simulink model "step2berevm"  (R2015a)
settings: Solver=ode45  StartTime=0.0  StopTime=1  RelTol=1e-3
values from neighbouring files (symbols this model uses):
  Dt = 1/(SampleRate*(N_in/N_out))    [DVBs2.m]    (also in DVBs2_2.m; Script.m)
  K_BCH = 51648    [DVBs2.m]    (also in DVBs2_2.m; Script.m)
  N_in = BBHEADER + DFL    [DVBs2.m]    (also in DVBs2_2.m; Script.m)
  Poly_ampl = polyfit(Xampl_0,DPDampl_0,PolyOrder)    [step1func.m]
  Poly_phase = polyfit(Xampl_0,DPDphase_0,PolyOrder)    [step1func.m]
  roll_off = 0.25    [DVBs2.m]    (also in DVBs2_2.m; Script.m)
undefined symbols (not defined in the file or in its folder): gcbh, rcfiltgaincompat
libraries: commblkcod2 x4, commfilt2 x3, commutil2 x2, dsppolyfun x2, dspsigops x2, commsequence2 x2, commdigbbndam3 x2, commblkintrlv2 x2, commchan3 x1, commrflib2 x1, commrandsrc2 x1, commsink2 x1
settings Model: Creator=Study  LastModifiedBy=Наталья
settings DataIOCC: SignalLoggingSaveFormat=ModelDataLogs
settings DebuggingCC: FcnCallInpInsideContextMsg=UseLocalSettings
settings GRTTargetCC: CombineOutputUpdateFcns=off  GRTInterface=on

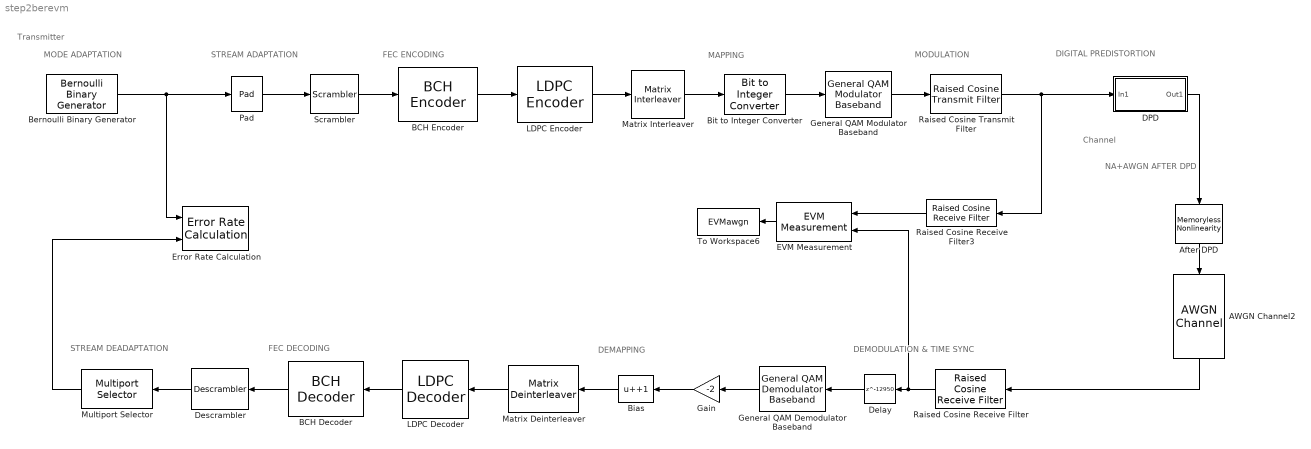
== system step2berevm ==
  note: DIGITAL PREDISTORTION
  note: DEMODULATION & TIME SYNC
  note: DEMAPPING
  note: FEC DECODING
  note: STREAM DEADAPTATION
  note: NA+AWGN
      | AFTER DPD
  note: Channel
  note: MODULATION
  note: MAPPING
  note: FEC ENCODING
  note: STREAM ADAPTATION
  note: MODE ADAPTATION
  note: Transmitter
  AWGN Channel2 : commchan3/AWGN Channel  InputProcessing=Columns as channels (frame based)  seed=67  noiseMode="Signal to noise ratio  (SNR)"  EbNodB=10  EsNodB=10  SNRdB=SNR  bitsPerSym=1  Ps=0.2562  Tsym=1  variance=1
  After DPD : commrflib2/Memoryless Nonlinearity  model_select=Saleh model  linGaindB=0  GindB=0  iip3=30  am2pm=10  LPwrLimAMPM=10  UPwrLimAMPM=inf  amam=AM_AM  ampm=AM_PM  x=[8.1081 1.5413 6.5202 -0.0718]  y=[4.6645 2.0965 10.88 -0.003]  p=0.5  GoutdB=0  vsat=1
  BCH Decoder : commblkcod2/BCH Decoder  n=N_BCH  k=K_BCH  specShortening=off  shortenedK=5  specGenPoly=on  genPoly=BCHGeneratorPoly  specPrimPoly=on  prPoly=BCHPrimitivePoly  specDisableGenCheck=off  specPuncture=off  punctVec=[ones(8,1); zeros(2,1)]  specErasurePort=off  showNumErr=off
  BCH Encoder : commblkcod2/BCH Encoder  n=N_BCH  k=K_BCH  specShortening=off  shortenedK=5  specGenPoly=on  genPoly=BCHGeneratorPoly  specPrimPoly=on  prPoly=BCHPrimitivePoly  specDisableGenCheck=off  specPuncture=off  punctVec=[ones(8,1); zeros(2,1)]
  Bernoulli Binary Generator : commrandsrc2/Bernoulli Binary Generator  P=0.5  seed=61  Ts=Dt  frameBased=on  sampPerFrame=N_in  orient=off  outDataType=double
  Bias : Bias  Bias=+1
  Bit to Integer Converter : commutil2/Bit to Integer Converter  nbits=NMOD  bitOrder=MSB first  signedOutputValues=Unsigned  outDtype=Inherit via internal rule  outDtypeSigned=Inherit via internal rule
  DPD : Subsystem
  Delay : Delay  DelayLength=12950  InitialCondition=0  InputProcessing=Columns as channels (frame based)
  Descrambler : commsequence2/Descrambler  M=2  poly=[1 0 0 0 0 0 0 0 0 0 0 0 0 0 1 1]  iniStaSource=Dialog Parameter  ini_sta=[1 0 0 1 0 1 0 1 0 0 0 0 0 0 0]  resetViaPort=off
  EVM Measurement : commutil2/EVM Measurement  normMethod=Average reference signal power  averagePower=1  peakPower=1  maxOrMinOut=off  percentileOut=off  percentileVal=95  nSym=off
  Error Rate Calculation : commsink2/Error Rate Calculation  N=N_in  st_delay=100  cp_mode=Entire frame  subframe=[]  PMode=Workspace  WsName=BERawgn  RsMode2=off  stop=off  numErr=100  maxBits=1e6
  Gain : Gain  Gain=-2
  General QAM Demodulator Baseband : commdigbbndam3/General QAM Demodulator Baseband  SigCon=apsk32  OutType=Bit  DecType=Hard decision  VarSource=Dialog  Variance=1  outDtypeBit=Inherit via internal rule  outDtype=Inherit via internal rule  roundingMode=Floor  overflowMode=Wrap  sigConstWordLen=16  accum1WordLen=32  accum1FracLen=30  prodInWordLen=32  prodInFracLen=30  prodOutWordLen=32  prodOutFracLen=30  accum2WordLen=32  accum2FracLen=30  accum3WordLen=32  accum3FracLen=30  nsiWordLen=32  nsiFracLen=30  invn0WordLen=16  invn0FracLen=8  outputWordLen=32  outputFracLen=30
  General QAM Modulator Baseband : commdigbbndam3/General QAM Modulator Baseband  SigCon=apsk32  outDtype=double  outWordLen=16  outUDDataType=sfix(16)  outFracLenMode=Best precision  outFracLen=15
  LDPC Decoder : commblkcod2/LDPC Decoder  ParityCheckMat=H  OutputFmt=Information part  DecisionType=Hard decision  OutputDataType=double  NumIter=50  DoParityCheck=on  OutputNumIter=off  OutputFinalChecks=off
  LDPC Encoder : commblkcod2/LDPC Encoder  ParityCheckMat=H
  Matrix Deinterleaver : commblkintrlv2/Matrix Deinterleaver  Nrows=Numofcols  Ncols=Numofrows
  Matrix Interleaver : commblkintrlv2/Matrix Interleaver  Nrows=Numofcols  Ncols=Numofrows
  Multiport Selector : dspindex/Multiport Selector  rowsOrCols=Rows  idxCellArray=[1:N_in]  idxErrMode=Clip Index
  Pad : dspsigops/Pad  padAlong=Columns  dimsToPad=1  valSrc=Specify via dialog  padVal=0  spec=Output size  padNumOutRowsSpecMethod=User-specified  numOutRows=K_BCH  padNumOutColsSpecMethod=User-specified  numOutCols=1  isVarDimsMode=off  padBeginning=0  padEnd=0  outSizeMode=User-specified  outSize=1  padSigAt=End  trunc_flag=None  roundingMode=Floor  overflowMode=off  truncOrWrapMode=Truncate  wrap_flag=None
  Raised Cosine Receive Filter : commfilt2/Raised Cosine Receive Filter  filtType=Square root  N=8  filtSpan=2*(10)/2  currentFiltSpan=2*(10)/2  D=(2*(10)/2)/2  R=roll_off  sampMode=Mute  saveAsFlag=0  rateMode=Downsampling  downFactor=8  downOffset=0  framing=Enforce single-rate processing  InputProcessing=Columns as channels (frame based)  checkGain=Normalized  filterGain=rcfiltgaincompat(gcbh)  checkCoeff=off  variableName=rcRxFilt  launchFVT=off  roundingMode=Floor  overflowMode=off
  Raised Cosine Receive Filter3 : commfilt2/Raised Cosine Receive Filter  filtType=Square root  N=8  filtSpan=2*(10)/2  currentFiltSpan=2*(10)/2  D=(2*(10)/2)/2  R=roll_off  sampMode=Mute  saveAsFlag=0  rateMode=Downsampling  downFactor=8  downOffset=0  framing=Enforce single-rate processing  InputProcessing=Columns as channels (frame based)  checkGain=Normalized  filterGain=rcfiltgaincompat(gcbh)  checkCoeff=off  variableName=rcRxFilt3  launchFVT=off  roundingMode=Floor  overflowMode=off
  Raised Cosine Transmit Filter : commfilt2/Raised Cosine Transmit Filter  filtType=Square root  filtSpan=2*(10)/2  currentFiltSpan=2*(10)/2  D=(2*(10)/2)/2  R=roll_off  sampMode=Mute  saveAsFlag=0  N=8  framing=Enforce single-rate processing  InputProcessing=Columns as channels (frame based)  checkGain=Normalized  filterGain=rcfiltgaincompat(gcbh)  checkCoeff=off  variableName=rcTxFilt  launchFVT=off  roundingMode=Floor  overflowMode=off
  Scrambler : commsequence2/Scrambler  M=2  poly=[1 0 0 0 0 0 0 0 0 0 0 0 0 0 1 1]  iniStaSource=Dialog Parameter  ini_sta=[1 0 0 1 0 1 0 1 0 0 0 0 0 0 0]  resetViaPort=off
  To Workspace6 : ToWorkspace  VariableName=EVMawgn  SampleTime=-1
      settings: Save2DSignal=2-D array (concatenate along first dimension)
  wires:
  Bernoulli Binary Generator/1 -> Error Rate Calculation/1, Pad/1
  Scrambler/1 -> BCH Encoder/1
  BCH Encoder/1 -> LDPC Encoder/1
  Pad/1 -> Scrambler/1
  Matrix Interleaver/1 -> Bit to Integer Converter/1
  Bit to Integer Converter/1 -> General QAM Modulator Baseband/1
  LDPC Encoder/1 -> Matrix Interleaver/1
  General QAM Modulator Baseband/1 -> Raised Cosine Transmit Filter/1
  General QAM Demodulator Baseband/1 -> Gain/1
  Gain/1 -> Bias/1
  Bias/1 -> Matrix Deinterleaver/1
  Matrix Deinterleaver/1 -> LDPC Decoder/1
  LDPC Decoder/1 -> BCH Decoder/1
  BCH Decoder/1 -> Descrambler/1
  Descrambler/1 -> Multiport Selector/1
  Delay/1 -> General QAM Demodulator Baseband/1
  Multiport Selector/1 -> Error Rate Calculation/2
  AWGN Channel2/1 -> Raised Cosine Receive Filter/1
  Raised Cosine Receive Filter/1 -> EVM Measurement/2, Delay/1
  After DPD/1 -> AWGN Channel2/1
  Raised Cosine Transmit Filter/1 -> Raised Cosine Receive Filter3/1, DPD/1(In1)
  EVM Measurement/1 -> To Workspace6/1
  Raised Cosine Receive Filter3/1 -> EVM Measurement/1
  DPD/1(Out1) -> After DPD/1

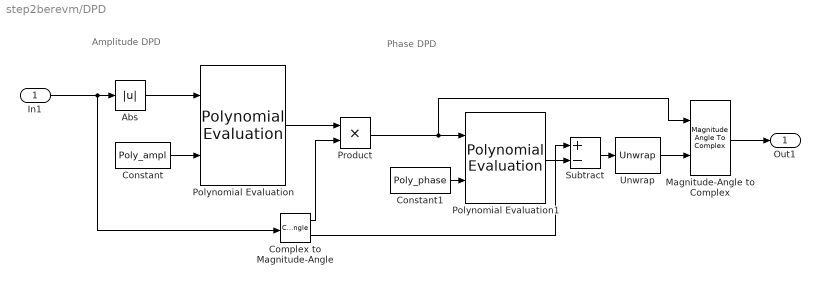
== system step2berevm/DPD ==
  note: Phase DPD
  note: Amplitude DPD
  In1 : Inport
  Abs : Abs
  Complex to Magnitude-Angle : ComplexToMagnitudeAngle
  Constant : Constant  Value=Poly_ampl  SampleTime=-1
  Constant1 : Constant  Value=Poly_phase
  Magnitude-Angle to Complex : MagnitudeAngleToComplex
  Polynomial Evaluation : dsppolyfun/Polynomial Evaluation  useConstCoeffs=off  constCoeffs=[5 4 3 2 1]
  Polynomial Evaluation1 : dsppolyfun/Polynomial Evaluation  useConstCoeffs=off  constCoeffs=[5 4 3 2 1]
  Product : Product
  Subtract : Sum  Inputs=+-
  Unwrap : dspsigops/Unwrap  tol=pi  InputProcessing=Columns as channels (frame based)  running=off
  Out1 : Outport
  wires:
  Magnitude-Angle to Complex/1 -> Out1/1
  Unwrap/1 -> Magnitude-Angle to Complex/2
  Constant/1 -> Polynomial Evaluation/2
  Polynomial Evaluation/1 -> Product/1
  In1/1 -> Complex to Magnitude-Angle/1, Abs/1
  Abs/1 -> Polynomial Evaluation/1
  Product/1 -> Magnitude-Angle to Complex/1, Polynomial Evaluation1/1
  Constant1/1 -> Polynomial Evaluation1/2
  Polynomial Evaluation1/1 -> Subtract/2
  Complex to Magnitude-Angle/1 -> Product/2
  Subtract/1 -> Unwrap/1
  Complex to Magnitude-Angle/2 -> Subtract/1
